simulink model "sim_switch_hover_vol"  (R2020b)
settings: Solver=VariableStepAuto  StartTime=0.0  StopTime=T  MaxStep=MaxStep  RelTol=RelTol
values from neighbouring files (symbols this model uses):
  a = 8000    [switch_hovering_vol.m]
  b = 15000    [switch_hovering_vol.m]
  controlleur = struct('kap',2.0,                       'kad',2.0,                       'kpp',1.0,                       'kpd',1.0,                       'k_delta',1.0,                       'u_barre',u_barre,                       'M_k',M_k,                       'skew_sym_d_etoile',skew_sym_d_etoile,                       'd_etoile', d_etoile                       )    [generateContolleur_hover.m]    (also in switch_hovering_vol.m = generateContolleur_hover(drone))
  controlleur_vol = generateContolleur(drone)    [switch_hovering_vol.m]
  drone = generateDarko()    [switch_hovering_vol.m]
  f_initial = drone.MASS*drone.G    [switch_hovering_vol.m]
  J = 200    [switch_hovering_vol.m]
  K_complet = [K(:,1:6), [0;0;0;0], K(:,7:12)]    [switch_hovering_vol.m]
  position_cible = [300; 300; 300]    [switch_hovering_vol.m]
  q_d_initial = ToQuaternion(yaw_d, pitch_d, roll_d)    [switch_hovering_vol.m]
  rule = 1    [switch_hovering_vol.m]
  S_complet = [S(1:6,1:6), zeros(6,1), S(1:6,7:12); zeros(1,13); S(7:12,1:6), zeros(6,1), S(7:12,7:12)]    [switch_hovering_vol.m]
  speed = 20    [switch_hovering_vol.m]
  T = 80    [switch_hovering_vol.m]
  u_eq_hover = drone.G*drone.MASS/(2*drone.Fb(1,1)) * [1;1;0;0]    [switch_hovering_vol.m]
  x0 = [p_initial; v_initial; q_initial; omega_initial; s]    [switch_hovering_vol.m]
  x_eq_hover = [[0; 0; 0]; [0; 0; 0]; [1/sqrt(2); 0; -1/sqrt(2);0]; [0; 0; 0]]    [switch_hovering_vol.m]
libraries: simulink_extras x6, simulink x3, pid_lib x1, sharedtransform x1
(part 2 of 2)

== matlab function sim_switch_hover_vol/Controlleur_vol_NL/Speed control ==
  data: speed input; x input; T1pT2 output; controlleur_vol parameter; drone parameter; vb output; G_b output
function [T1pT2, vb, G_b]   = speed_control(speed, x, controlleur_vol, drone)
%#codegen 

% gravity
g = drone.G;
% vehicle mass
m = drone.MASS;
rho = drone.RHO;
% ws = drone.WINGSPAN;
% chord = drone.CHORD;
Swet = drone.WET_SURFACE;
Sdry = drone.DRY_SURFACE;
S = Swet + Sdry;

PHI_fv = drone.PHI(1:3,1:3);


% p = x(1:3);
v = x(4:6);
q  = x(7:10);
w = x(11:13);

eta = sqrt(norm(v)^2);
D = q2dcm(q);

vb = D'*v;
vbx = vb(1);
% vby = vb(2);
% vbz = vb(3);

G_b = D'*[0;0;g];

ay = drone.P_A2_CG(2);
py = drone.P_P2_CG(2);
die_c = drone.PHI(3,3);
Cd0 = drone.PHI(1,1);

Swet   = drone.WET_SURFACE;
Sdry   = drone.DRY_SURFACE;
Sp = pi*drone.PROP_RADIUS^2;
Thetam = drone.ELEVON_MEFFICIENCY(2);
% Thetaf = drone.ELEVON_FEFFICIENCY(2);
kf = drone.PROP_KP;
km = drone.PROP_KM;
S = Swet + Sdry;
rho    = drone.RHO;
phi_n  = drone.PHI_n;
chord  = drone.CHORD;
ws     = drone.WINGSPAN;
B = diag([ws; chord; ws]);
dR = drone.CENTRAGE ;
eta = sqrt( norm(v)^2 + phi_n*norm(B*w)^2 );

% T1pT2 = 1/(2*(1-(Swet/(4*Sp))*Cd0))*rho*S*eta*Cd0*vbx + G_b(1) + controlleur.kv * (speed - vb(1));
 T1pT2 = controlleur_vol.kv * (speed - vb(1));

== matlab function sim_switch_hover_vol/Controlleur_vol_NL/vecteur de commande ==
  data: cmd_vect input; u output
function u = fcn(cmd_vect)

T1pT2 = cmd_vect(1);
T1mT2 = cmd_vect(2);
d1pd2 = cmd_vect(3);
d1md2 = cmd_vect(4);

u = [1/2*(T1pT2 + T1mT2); 1/2*(T1pT2 - T1mT2); 1/2*(d1pd2 + d1md2); 1/2*(d1pd2 - d1md2)];

== matlab function sim_switch_hover_vol/MATLAB Function3 ==
  data: u input; y output
function y = fcn(u)
%#codegen

y = norm(u);

== matlab function sim_switch_hover_vol/Controlleur_vol_NL/Select ==
  data: x input; vbx output
function vbx = select(x)
v = x(4:6);
q  = x(7:10);
D = q2dcm(q);

vb = D'*v;
vbx = vb(1);

== matlab function sim_switch_hover_vol/Controlleur_hover_NL/Satutation des commandes/convert ==
  data: u input; w1 output; drone parameter; w2 output; d1 output; d2 output
function [w1, w2, d1, d2] = convert(u, drone)
%#codegen
kf = drone.PROP_KP;

T1 = max(u(1),0);
T2 = max(u(2),0);
d1_T1 = u(3);
d2_T2 = u(4);

w1 = sqrt(T1/kf);
w2 = sqrt(T2/kf);
d1 = d1_T1/T1;
d2 = d2_T2/T2;

== matlab function sim_switch_hover_vol/Controlleur_hover_NL/Contoller state/MATLAB Function ==
  data: n output; q input; mismatch output; cor output
function [n, mismatch, cor] = fcn(q)
%#codegen
n = norm(q);
mismatch = 1-norm(q);
cor = mismatch*q;

== matlab function sim_switch_hover_vol/Controlleur_vol_NL/Satutation des commandes/convert ==
  data: u input size=4; w1 output; drone parameter; w2 output; d1 output; d2 output
function [w1, w2, d1, d2] = convert(u, drone)
%#codegen
kf = drone.PROP_KP;

T1 = max(u(1),0);
T2 = max(u(2),0);
d1 = u(3);
d2 = u(4);

w1 = sqrt(T1/kf);
w2 = sqrt(T2/kf);

== matlab function sim_switch_hover_vol/Controlleur_hover_NL/Contoller state/Quaternion dyn ==
  data: q input; q_dot output; omega input
function q_dot = q_dyn(q, omega)
%#codegen

eta = q(1);
eps = q(2:4);

A = [-eps';  eta*eye(3)+skew_sym(eps)];
q_dot = 1/2*A*omega;
